simulink model "hydrofoil_sim_unified"  (R2024b)
settings: Solver=VariableStepAuto  StartTime=0.0  StopTime=20  FixedStep=0.05  MaxStep=0.2  RelTol=1e-3
values from neighbouring files (symbols this model uses):
  AfoilA = 0.046    [model_parameters.m]
  AfoilFP = 0.048    [model_parameters.m]
  AfoilFS = 0.048    [model_parameters.m]
  alpha0012 = data0012(:,1)    [model_parameters.m]
  alpha63412wing = data63412wing(:,1)    [model_parameters.m]
  cd0012 = data0012(:,3)    [model_parameters.m]
  cdi63412wing = data63412wing(:,4)    [model_parameters.m]
  cdv63412wing = data63412wing(:,5)    [model_parameters.m]
  cl63412wing = data63412wing(:,3)    [model_parameters.m]
  cm63412wing = data63412wing(:,9)    [model_parameters.m]
  csA = 0.1    [model_parameters.m]
  csF = 0.08    [model_parameters.m]
  deltat = 1/100    (= 0.01)    [model_parameters.m]
  foilA_ARM = [-dxa, dya, dza]    [model_parameters.m]
  foilFP_ARM = [dxf, -dyf, dzf]    [model_parameters.m]
  foilFS_ARM = [dxf, dyf, dzf]    [model_parameters.m]
  g = 9.81    [model_parameters.m]
  LAd = 0.08*pi*(0.8)^3/64    (= 0.0020106192983)    [model_parameters.m]
  LFPd = integral(fpint, foilFP_ARM(2)-0.4, foilFP_ARM(2)+0.4)    [model_parameters.m]
  LFSd = integral(fsint, foilFS_ARM(2)-0.4, foilFS_ARM(2)+0.4)    [model_parameters.m]
  M_RB_1 = inv(M_RB)    [dimensionalize_model.m]    (also in model_parameters.m = M_RB^(-1))
  MAC_A = 0.08    [model_parameters.m]
  MAC_FP = 0.08    [model_parameters.m]
  MAC_FS = 0.08    [model_parameters.m]
  mass = 215    [dimensionalize_model.m]    (also in model_parameters.m)
  propwake = 0.05    [model_parameters.m]
  psd_acc = (9.81*60*1e-6)^2    (= 3.4644996e-07)    [model_parameters.m]
  psd_gyro = (1.222*1e-4)^2    (= 1.493284e-08)    [model_parameters.m]
  r_g = [0; 0; 0]    [dimensionalize_model.m]    (also in model_parameters.m = [xg, yg, zg])
  rho = 1024.8    [model_parameters.m]
  seed_accX = 1324    [model_parameters.m]
  seed_accZ = 1432    [model_parameters.m]
  seed_gps = 4321    [model_parameters.m]
  seed_gyroX = 243251    [model_parameters.m]
  seed_gyroY = 3124234    [model_parameters.m]
  seed_pitch = 7568    [model_parameters.m]
  seed_roll = 35642    [model_parameters.m]
  seed_sonar = 1234    [model_parameters.m]
  setpoint_signals = setpoints.preview    [model_parameters.m]
  sonar_position = [dxf+0.5; 0; -0.1]    [model_parameters.m]
  spanA = 0.76    [model_parameters.m]
  spanFP = 0.76    [model_parameters.m]
  spanFS = 0.76    [model_parameters.m]
  tA = 0.12*0.08    (= 0.0096)    [model_parameters.m]
  tFP = 0.12*0.08    (= 0.0096)    [model_parameters.m]
  tFS = 0.12*0.08    (= 0.0096)    [model_parameters.m]
  usted = 7    [model_parameters.m]
  var_angle = deg2rad(0.2)^2    [model_parameters.m]
  var_gps = 0.05^2    (= 0.0025)    [model_parameters.m]
  var_sonar = 0.002^2    (= 4e-06)    [model_parameters.m]
  wagC1 = 0.165    [model_parameters.m]
  wagC2 = 0.335    [model_parameters.m]
  wage1 = 0.0455*(usted/(MAC_FP/2))    (= 7.9625)    [model_parameters.m]
  wage2 = 0.3*(usted/(MAC_FP/2))    (= 52.5)    [model_parameters.m]
  wave_data = struct('amplitude',0,'omega',0,'wavenumber',0,'phase',0,'direction',0)    [model_parameters.m]
  zpr = dza    (= 0.96)    [model_parameters.m]
undefined symbols (not defined in the file or in its folder): act_lims, actuation_tau, bA, bB, bC, bD, dLTI_array_IDP, dLTI_array_IP, Ka, Klqid, magnitude, PredictionHorizon, set, Ts_reference_preview, V_vals
libraries: mssSimulink x15, mpclib x10, simulink x6, simulink_extras x5, cstblocks x4, matrix_library x3, slpidlib x1
(part 2 of 3)

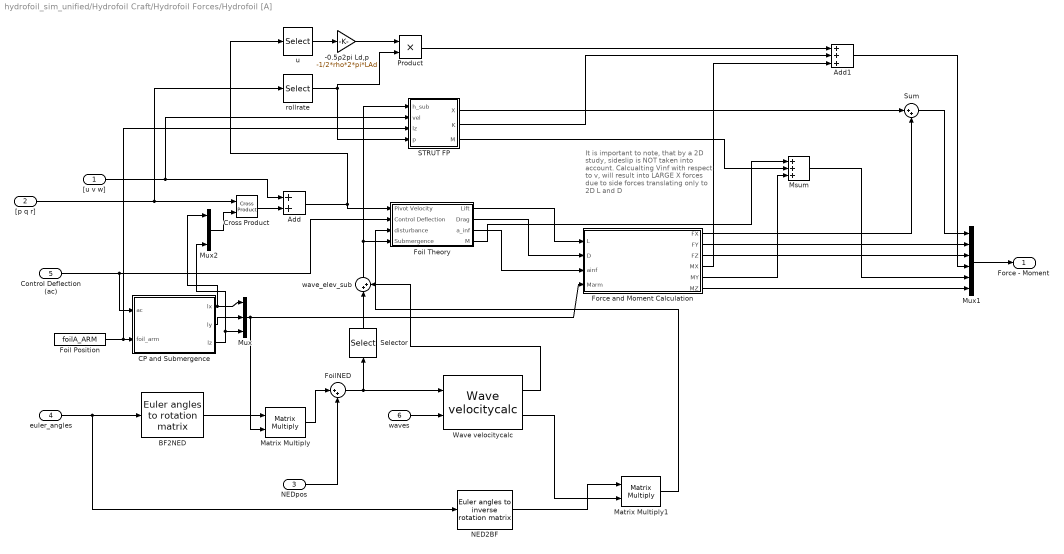
== system hydrofoil_sim_unified/Hydrofoil Craft/Hydrofoil Forces/Hydrofoil [A] ==
  note: It is important to note,
      | that by a 2D study, sideslip
      | is NOT taken into account.
      | Calcualting Vinf with respect
      | to v, will result into LARGE X
      | forces due to side forces translating
      | only to 2D L and D
  "[u v w]" : Inport
  "[p q r]" : Inport  Port=2
  NEDpos : Inport  Port=3
  euler_angles : Inport  Port=4
  Control Deflection (ac) : Inport  Port=5
  waves : Inport  Port=6
  -0.5ρ2pi Ld,p : Gain  Gain=-1/2*rho*2*pi*LAd
  Add : Sum
  Add1 : Sum  Inputs=+++
  BF2NED : mssSimulink/Modelling/Kinematics/Euler angles to rotation matrix
  CP and Submergence : MATLAB Function  TreatAsAtomicUnit=on
  Cross Product : matrix_library/Cross Product
  Foil Position : Constant  Value=foilA_ARM
  Foil Theory : Subsystem
  FoilNED : Sum  Inputs=|++
  Force and Moment Calculation : MATLAB Function  TreatAsAtomicUnit=on
  Matrix Multiply : Product  Multiplication=Matrix(*)
  Matrix Multiply1 : Product  Multiplication=Matrix(*)
  Msum : Sum  Inputs=+++
  Mux : Mux  Inputs=3
  Mux1 : Mux  Inputs=6
  Mux2 : Mux  Inputs=3
  NED2BF : mssSimulink/Modelling/Kinematics/Euler angles to inverse rotation matrix
  Product : Product
  STRUT FP : Subsystem
  Selector : Selector  InputPortWidth=3  IndexOptions=Index vector (dialog)  Indices=[3]  OutputSizes=1
  Sum : Sum  Inputs=|++
  Wave velocitycalc : mssSimulink/Environment/Waves/Wave velocitycalc
  rollrate : Selector  InputPortWidth=3  IndexOptions=Index vector (dialog)  Indices=[1]  OutputSizes=1
  u : Selector  InputPortWidth=3  IndexOptions=Index vector (dialog)  Indices=[1]  OutputSizes=1
  wave_elev_sub : Sum  Inputs=|++
  Force - Moment : Outport
  wires:
  "[u v w]"/1 -> STRUT FP/2(vel), Add/1
  Cross Product/1 -> Add/2
  "[p q r]"/1 -> rollrate/1, Cross Product/1
  Control Deflection (ac)/1 -> Foil Theory/2(Control Deflection), CP and Submergence/1(ac)
  CP and Submergence/1(lx) -> Mux2/1, Mux/1
  CP and Submergence/2(ly) -> Mux/2
  CP and Submergence/3(lz) -> Mux2/3, Mux/3
  Mux/1 -> Matrix Multiply/2, Force and Moment Calculation/4(Marm)
  Force and Moment Calculation/2(FY) -> Mux1/2
  Force and Moment Calculation/3(FZ) -> Mux1/3
  Force and Moment Calculation/6(MZ) -> Mux1/6
  Mux1/1 -> Force - Moment/1
  Foil Position/1 -> STRUT FP/3(lz), CP and Submergence/2(foil_arm)
  euler_angles/1 -> NED2BF/1, BF2NED/1
  Add/1 -> u/1, Foil Theory/1(Pivot Velocity)
  Foil Theory/1(Lift) -> Force and Moment Calculation/1(L)
  Foil Theory/2(Drag) -> Force and Moment Calculation/2(D)
  Foil Theory/3(a_inf) -> Force and Moment Calculation/3(ainf)
  BF2NED/1 -> Matrix Multiply/1
  Matrix Multiply/1 -> FoilNED/1
  NEDpos/1 -> FoilNED/2
  FoilNED/1 -> Wave velocitycalc/1, Selector/1
  Sum/1 -> Mux1/1
  Force and Moment Calculation/1(FX) -> Sum/2
  STRUT FP/1(X) -> Sum/1
  STRUT FP/3(M) -> Msum/2
  Force and Moment Calculation/5(MY) -> Msum/3
  Msum/1 -> Mux1/5
  STRUT FP/2(K) -> Add1/2
  Force and Moment Calculation/4(MX) -> Add1/3
  Add1/1 -> Mux1/4
  Mux2/1 -> Cross Product/2
  rollrate/1 -> Product/2, STRUT FP/4(p)
  -0.5ρ2pi Ld,p/1 -> Product/1
  u/1 -> -0.5ρ2pi Ld,p/1
  Product/1 -> Add1/1
  Wave velocitycalc/1 -> wave_elev_sub/2
  Wave velocitycalc/2 -> Matrix Multiply1/2
  NED2BF/1 -> Matrix Multiply1/1
  wave_elev_sub/1 -> STRUT FP/1(h_sub), Foil Theory/4(Submergence)
  Selector/1 -> wave_elev_sub/1
  waves/1 -> Wave velocitycalc/2
  Matrix Multiply1/1 -> Foil Theory/3(disturbance)
  Foil Theory/4(M) -> Msum/1

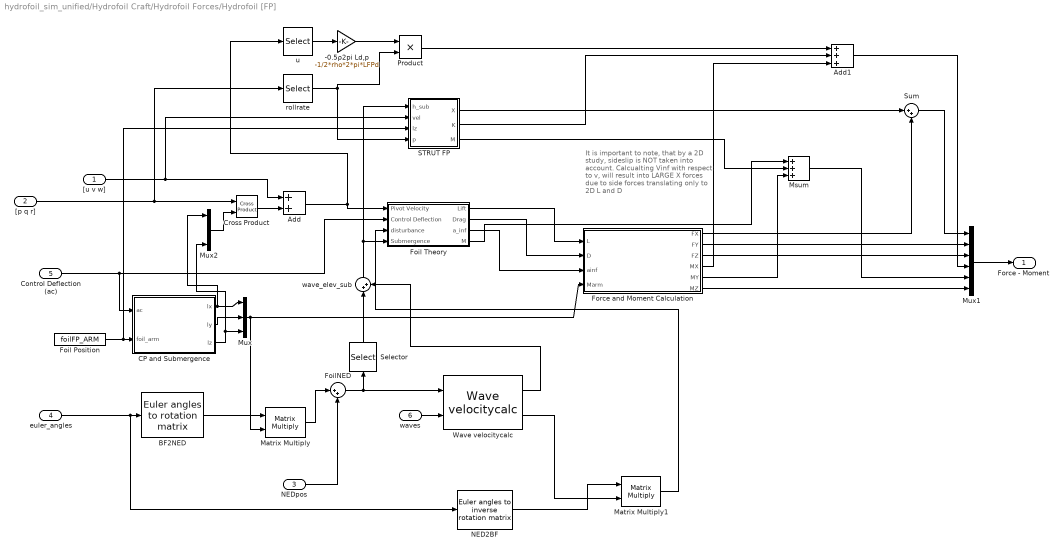
== system hydrofoil_sim_unified/Hydrofoil Craft/Hydrofoil Forces/Hydrofoil [FP] ==
  note: It is important to note,
      | that by a 2D study, sideslip
      | is NOT taken into account.
      | Calcualting Vinf with respect
      | to v, will result into LARGE X
      | forces due to side forces translating
      | only to 2D L and D
  "[u v w]" : Inport
  "[p q r]" : Inport  Port=2
  NEDpos : Inport  Port=3
  euler_angles : Inport  Port=4
  Control Deflection (ac) : Inport  Port=5
  waves : Inport  Port=6
  -0.5ρ2pi Ld,p : Gain  Gain=-1/2*rho*2*pi*LFPd
  Add : Sum
  Add1 : Sum  Inputs=+++
  BF2NED : mssSimulink/Modelling/Kinematics/Euler angles to rotation matrix
  CP and Submergence : MATLAB Function  TreatAsAtomicUnit=on
  Cross Product : matrix_library/Cross Product
  Foil Position : Constant  Value=foilFP_ARM
  Foil Theory : Subsystem
  FoilNED : Sum  Inputs=|++
  Force and Moment Calculation : MATLAB Function  TreatAsAtomicUnit=on
  Matrix Multiply : Product  Multiplication=Matrix(*)
  Matrix Multiply1 : Product  Multiplication=Matrix(*)
  Msum : Sum  Inputs=+++
  Mux : Mux  Inputs=3
  Mux1 : Mux  Inputs=6
  Mux2 : Mux  Inputs=3
  NED2BF : mssSimulink/Modelling/Kinematics/Euler angles to inverse rotation matrix
  Product : Product
  STRUT FP : Subsystem
  Selector : Selector  InputPortWidth=3  IndexOptions=Index vector (dialog)  Indices=[3]  OutputSizes=1
  Sum : Sum  Inputs=|++
  Wave velocitycalc : mssSimulink/Environment/Waves/Wave velocitycalc
  rollrate : Selector  InputPortWidth=3  IndexOptions=Index vector (dialog)  Indices=[1]  OutputSizes=1
  u : Selector  InputPortWidth=3  IndexOptions=Index vector (dialog)  Indices=[1]  OutputSizes=1
  wave_elev_sub : Sum  Inputs=|++
  Force - Moment : Outport
  wires:
  "[u v w]"/1 -> STRUT FP/2(vel), Add/1
  Cross Product/1 -> Add/2
  "[p q r]"/1 -> rollrate/1, Cross Product/1
  Control Deflection (ac)/1 -> Foil Theory/2(Control Deflection), CP and Submergence/1(ac)
  CP and Submergence/1(lx) -> Mux2/1, Mux/1
  CP and Submergence/2(ly) -> Mux/2
  CP and Submergence/3(lz) -> Mux2/3, Mux/3
  Mux/1 -> Matrix Multiply/2, Force and Moment Calculation/4(Marm)
  Force and Moment Calculation/2(FY) -> Mux1/2
  Force and Moment Calculation/3(FZ) -> Mux1/3
  Force and Moment Calculation/6(MZ) -> Mux1/6
  Mux1/1 -> Force - Moment/1
  Foil Position/1 -> STRUT FP/3(lz), CP and Submergence/2(foil_arm)
  euler_angles/1 -> NED2BF/1, BF2NED/1
  Add/1 -> u/1, Foil Theory/1(Pivot Velocity)
  Foil Theory/1(Lift) -> Force and Moment Calculation/1(L)
  Foil Theory/2(Drag) -> Force and Moment Calculation/2(D)
  Foil Theory/3(a_inf) -> Force and Moment Calculation/3(ainf)
  BF2NED/1 -> Matrix Multiply/1
  Matrix Multiply/1 -> FoilNED/1
  NEDpos/1 -> FoilNED/2
  FoilNED/1 -> Wave velocitycalc/1, Selector/1
  Sum/1 -> Mux1/1
  Force and Moment Calculation/1(FX) -> Sum/2
  STRUT FP/1(X) -> Sum/1
  STRUT FP/3(M) -> Msum/2
  Force and Moment Calculation/5(MY) -> Msum/3
  Msum/1 -> Mux1/5
  STRUT FP/2(K) -> Add1/2
  Force and Moment Calculation/4(MX) -> Add1/3
  Add1/1 -> Mux1/4
  Mux2/1 -> Cross Product/2
  rollrate/1 -> Product/2, STRUT FP/4(p)
  -0.5ρ2pi Ld,p/1 -> Product/1
  u/1 -> -0.5ρ2pi Ld,p/1
  Product/1 -> Add1/1
  waves/1 -> Wave velocitycalc/2
  Wave velocitycalc/1 -> wave_elev_sub/2
  NED2BF/1 -> Matrix Multiply1/1
  Wave velocitycalc/2 -> Matrix Multiply1/2
  Selector/1 -> wave_elev_sub/1
  wave_elev_sub/1 -> STRUT FP/1(h_sub), Foil Theory/4(Submergence)
  Matrix Multiply1/1 -> Foil Theory/3(disturbance)
  Foil Theory/4(M) -> Msum/1

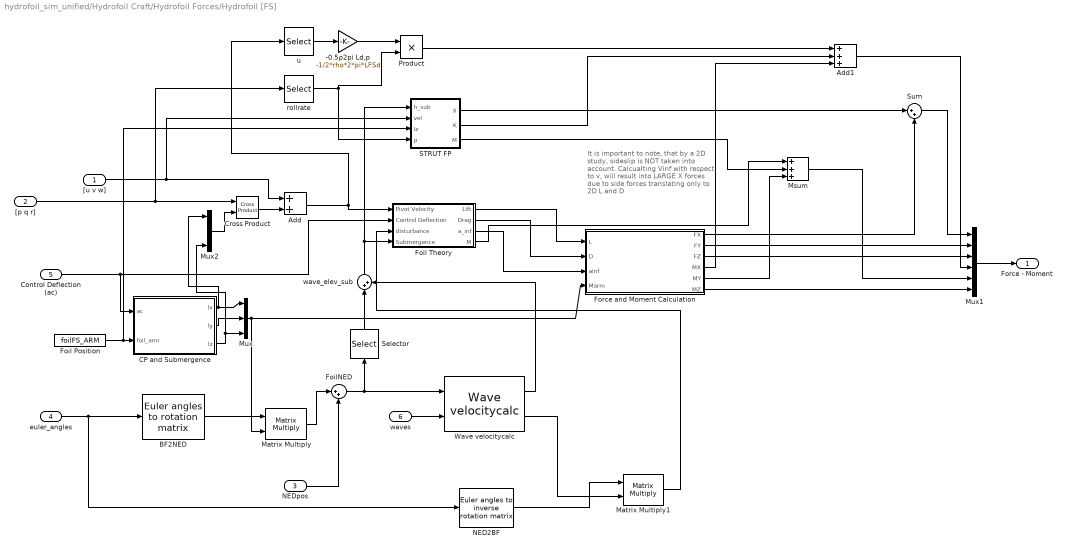
== system hydrofoil_sim_unified/Hydrofoil Craft/Hydrofoil Forces/Hydrofoil [FS] ==
  note: It is important to note,
      | that by a 2D study, sideslip
      | is NOT taken into account.
      | Calcualting Vinf with respect
      | to v, will result into LARGE X
      | forces due to side forces translating
      | only to 2D L and D
  "[u v w]" : Inport
  "[p q r]" : Inport  Port=2
  NEDpos : Inport  Port=3
  euler_angles : Inport  Port=4
  Control Deflection (ac) : Inport  Port=5
  waves : Inport  Port=6
  -0.5ρ2pi Ld,p : Gain  Gain=-1/2*rho*2*pi*LFSd
  Add : Sum
  Add1 : Sum  Inputs=+++
  BF2NED : mssSimulink/Modelling/Kinematics/Euler angles to rotation matrix
  CP and Submergence : MATLAB Function  TreatAsAtomicUnit=on
  Cross Product : matrix_library/Cross Product
  Foil Position : Constant  Value=foilFS_ARM
  Foil Theory : Subsystem
  FoilNED : Sum  Inputs=|++
  Force and Moment Calculation : MATLAB Function  TreatAsAtomicUnit=on
  Matrix Multiply : Product  Multiplication=Matrix(*)
  Matrix Multiply1 : Product  Multiplication=Matrix(*)
  Msum : Sum  Inputs=+++
  Mux : Mux  Inputs=3
  Mux1 : Mux  Inputs=6
  Mux2 : Mux  Inputs=3
  NED2BF : mssSimulink/Modelling/Kinematics/Euler angles to inverse rotation matrix
  Product : Product
  STRUT FP : Subsystem
  Selector : Selector  InputPortWidth=3  IndexOptions=Index vector (dialog)  Indices=[3]  OutputSizes=1
  Sum : Sum  Inputs=|++
  Wave velocitycalc : mssSimulink/Environment/Waves/Wave velocitycalc
  rollrate : Selector  InputPortWidth=3  IndexOptions=Index vector (dialog)  Indices=[1]  OutputSizes=1
  u : Selector  InputPortWidth=3  IndexOptions=Index vector (dialog)  Indices=[1]  OutputSizes=1
  wave_elev_sub : Sum  Inputs=|++
  Force - Moment : Outport
  wires:
  "[u v w]"/1 -> STRUT FP/2(vel), Add/1
  Cross Product/1 -> Add/2
  "[p q r]"/1 -> rollrate/1, Cross Product/1
  Control Deflection (ac)/1 -> Foil Theory/2(Control Deflection), CP and Submergence/1(ac)
  CP and Submergence/1(lx) -> Mux2/1, Mux/1
  CP and Submergence/2(ly) -> Mux/2
  CP and Submergence/3(lz) -> Mux2/3, Mux/3
  Mux/1 -> Matrix Multiply/2, Force and Moment Calculation/4(Marm)
  Force and Moment Calculation/2(FY) -> Mux1/2
  Force and Moment Calculation/3(FZ) -> Mux1/3
  Force and Moment Calculation/6(MZ) -> Mux1/6
  Mux1/1 -> Force - Moment/1
  Foil Position/1 -> STRUT FP/3(lz), CP and Submergence/2(foil_arm)
  euler_angles/1 -> NED2BF/1, BF2NED/1
  Add/1 -> u/1, Foil Theory/1(Pivot Velocity)
  Foil Theory/1(Lift) -> Force and Moment Calculation/1(L)
  Foil Theory/2(Drag) -> Force and Moment Calculation/2(D)
  Foil Theory/3(a_inf) -> Force and Moment Calculation/3(ainf)
  BF2NED/1 -> Matrix Multiply/1
  Matrix Multiply/1 -> FoilNED/1
  NEDpos/1 -> FoilNED/2
  FoilNED/1 -> Selector/1, Wave velocitycalc/1
  Sum/1 -> Mux1/1
  Force and Moment Calculation/1(FX) -> Sum/2
  STRUT FP/1(X) -> Sum/1
  STRUT FP/3(M) -> Msum/2
  Force and Moment Calculation/5(MY) -> Msum/3
  Msum/1 -> Mux1/5
  STRUT FP/2(K) -> Add1/2
  Force and Moment Calculation/4(MX) -> Add1/3
  Add1/1 -> Mux1/4
  Mux2/1 -> Cross Product/2
  rollrate/1 -> Product/2, STRUT FP/4(p)
  -0.5ρ2pi Ld,p/1 -> Product/1
  u/1 -> -0.5ρ2pi Ld,p/1
  Product/1 -> Add1/1
  Wave velocitycalc/1 -> wave_elev_sub/2
  Wave velocitycalc/2 -> Matrix Multiply1/2
  NED2BF/1 -> Matrix Multiply1/1
  Selector/1 -> wave_elev_sub/1
  wave_elev_sub/1 -> STRUT FP/1(h_sub), Foil Theory/4(Submergence)
  waves/1 -> Wave velocitycalc/2
  Matrix Multiply1/1 -> Foil Theory/3(disturbance)
  Foil Theory/4(M) -> Msum/1

== system hydrofoil_sim_unified/sense/sonar/sensor ==
  environment : Inport
  position : Inport  Port=2
  angles : Inport  Port=3
  sonar_pos : Inport  Port=4
  BF2NED : mssSimulink/Modelling/Kinematics/Euler angles to rotation matrix
  Product : Product  Multiplication=Matrix(*)
  Sum : Sum  Inputs=|++
  Sum1 : Sum  Inputs=|++
  Wave velocitycalc : mssSimulink/Environment/Waves/Wave velocitycalc
  get_hs : MATLAB Function  TreatAsAtomicUnit=on
  sonar_height : Outport
  wires:
  environment/1 -> Wave velocitycalc/2
  position/1 -> get_hs/1(positionCG), Sum/1
  angles/1 -> get_hs/2(euler_angles), BF2NED/1
  sonar_pos/1 -> get_hs/3(sonar_position)
  Sum/1 -> Wave velocitycalc/1
  Wave velocitycalc/1 -> Sum1/1
  get_hs/1(h_s) -> Sum1/2
  Sum1/1 -> sonar_height/1
  BF2NED/1 -> Product/1
  get_hs/2(d_s) -> Product/2
  Product/1 -> Sum/2

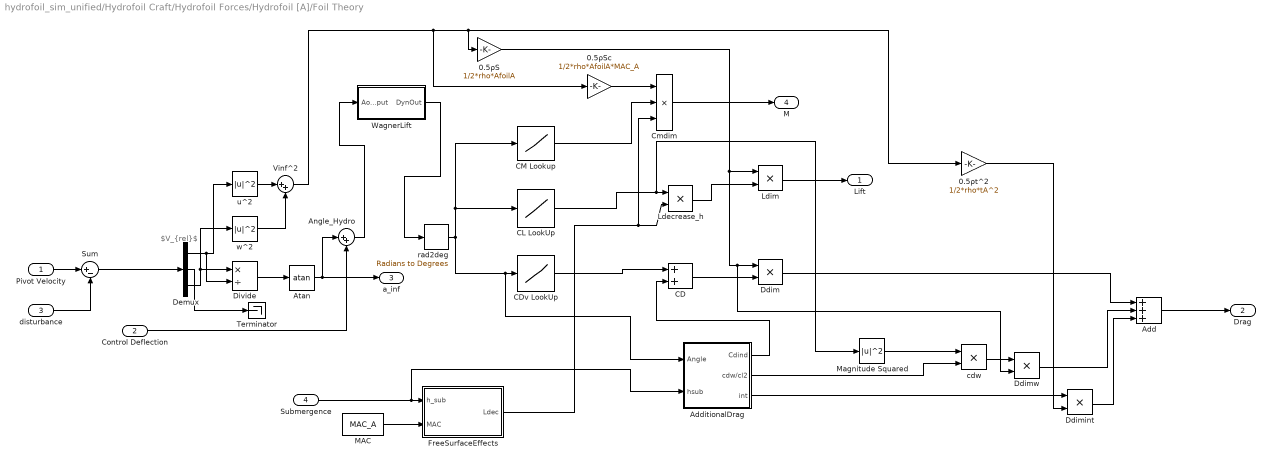
== system hydrofoil_sim_unified/Hydrofoil Craft/Hydrofoil Forces/Hydrofoil [A]/Foil Theory ==
  note: $V_{rel}$
  Pivot Velocity : Inport
  Control Deflection : Inport  Port=2
  disturbance : Inport  Port=3
  Submergence : Inport  Port=4
  0.5ρS : Gain  Gain=1/2*rho*AfoilA
  0.5ρSc : Gain  Gain=1/2*rho*AfoilA*MAC_A
  0.5ρt^2 : Gain  Gain=1/2*rho*tA^2
  Add : Sum  Inputs=+++
  AdditionalDrag : Subsystem
  Angle_Hydro : Sum  Inputs=|++
  Atan : Trigonometry  Operator=atan
  CD : Sum
  CDv LookUp : Lookup_n-D  NumberOfTableDimensions=1  BreakpointsForDimension1=alpha63412wing  Table=cdv63412wing  InternalRulePriority=Speed  RndMeth=Simplest
  CL LookUp : Lookup_n-D  NumberOfTableDimensions=1  BreakpointsForDimension1=alpha63412wing  Table=cl63412wing  InternalRulePriority=Speed  RndMeth=Simplest
  CM Lookup : Lookup_n-D  NumberOfTableDimensions=1  BreakpointsForDimension1=alpha63412wing  Table=cm63412wing  InternalRulePriority=Speed  RndMeth=Simplest
  Cmdim : Product  Inputs=3
  Ddim : Product
  Ddimint : Product
  Ddimw : Product
  Demux : Demux  Outputs=3
  Divide : Product  Inputs=*/
  FreeSurfaceEffects : MATLAB Function  TreatAsAtomicUnit=on
  Ldecrease_h : Product
  Ldim : Product
  MAC : Constant  Value=MAC_A
  Magnitude Squared : Math  Operator=magnitude^2
  Sum : Sum  Inputs=|+-
  Terminator : Terminator
  Vinf^2 : Sum  Inputs=|++
  WagnerLift : Subsystem
  cdw : Product
  rad2deg : simulink_extras/Transformations/Radians to Degrees
  u^2 : Math  Operator=magnitude^2
  w^2 : Math  Operator=magnitude^2
  Lift : Outport
  Drag : Outport  Port=2
  a_inf : Outport  Port=3
  M : Outport  Port=4
  wires:
  rad2deg/1 -> AdditionalDrag/1(Angle), CDv LookUp/1, CM Lookup/1, CL LookUp/1
  Demux/3 -> w^2/1, Divide/1
  Vinf^2/1 -> 0.5ρSc/1, 0.5ρS/1, 0.5ρt^2/1
  w^2/1 -> Vinf^2/2
  Demux/1 -> u^2/1, Divide/2
  Atan/1 -> a_inf/1, Angle_Hydro/1
  0.5ρS/1 -> Ddimw/2, Ddim/1, Ldim/1
  u^2/1 -> Vinf^2/1
  Divide/1 -> Atan/1
  Control Deflection/1 -> Angle_Hydro/2
  Demux/2 -> Terminator/1
  Ldim/1 -> Lift/1
  Sum/1 -> Demux/1
  disturbance/1 -> Sum/2
  Pivot Velocity/1 -> Sum/1
  Submergence/1 -> AdditionalDrag/2(hsub), FreeSurfaceEffects/1(h_sub)
  MAC/1 -> FreeSurfaceEffects/2(MAC)
  FreeSurfaceEffects/1(Ldec) -> Cmdim/3, Ldecrease_h/2
  CL LookUp/1 -> Magnitude Squared/1, Ldecrease_h/1
  Ldecrease_h/1 -> Ldim/2
  CDv LookUp/1 -> CD/1
  CD/1 -> Ddim/2
  AdditionalDrag/1(Cdind) -> CD/2
  Ddim/1 -> Add/1
  Magnitude Squared/1 -> cdw/1
  AdditionalDrag/2(cdw/cl2) -> cdw/2
  cdw/1 -> Ddimw/1
  Ddimw/1 -> Add/2
  AdditionalDrag/3(int) -> Ddimint/1
  Add/1 -> Drag/1
  0.5ρt^2/1 -> Ddimint/2
  Ddimint/1 -> Add/3
  Angle_Hydro/1 -> WagnerLift/1(AoA Input)
  CM Lookup/1 -> Cmdim/2
  0.5ρSc/1 -> Cmdim/1
  Cmdim/1 -> M/1
  WagnerLift/1(DynOut) -> rad2deg/1

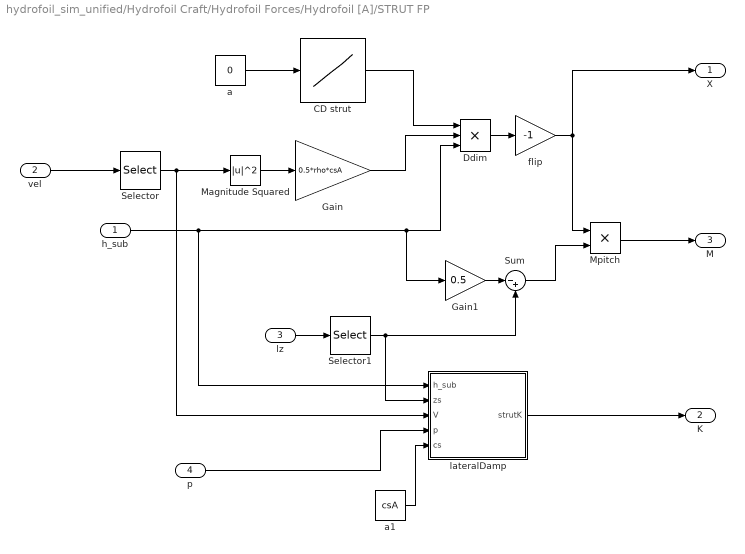
== system hydrofoil_sim_unified/Hydrofoil Craft/Hydrofoil Forces/Hydrofoil [A]/STRUT FP ==
  h_sub : Inport
  vel : Inport  Port=2
  lz : Inport  Port=3
  p : Inport  Port=4
  CD strut : Lookup_n-D  NumberOfTableDimensions=1  BreakpointsForDimension1=alpha0012  Table=cd0012  InternalRulePriority=Speed  RndMeth=Simplest
  Ddim : Product  Inputs=3
  Gain : Gain  Gain=0.5*rho*csA
  Gain1 : Gain  Gain=0.5
  Magnitude Squared : Math  Operator=magnitude^2
  Mpitch : Product
  Selector : Selector  InputPortWidth=3  IndexOptions=Index vector (dialog)  Indices=[1]  OutputSizes=1
  Selector1 : Selector  InputPortWidth=3  IndexOptions=Index vector (dialog)  Indices=[3]  OutputSizes=1
  Sum : Sum  Inputs=|-+
  a : Constant  Value=0
  a1 : Constant  Value=csA
  flip : Gain  Gain=-1
  lateralDamp : MATLAB Function  TreatAsAtomicUnit=on
  X : Outport
  K : Outport  Port=2
  M : Outport  Port=3
  wires:
  vel/1 -> Selector/1
  Selector/1 -> Magnitude Squared/1, lateralDamp/3(V)
  Magnitude Squared/1 -> Gain/1
  a/1 -> CD strut/1
  CD strut/1 -> Ddim/1
  Gain/1 -> Ddim/2
  h_sub/1 -> lateralDamp/1(h_sub), Ddim/3, Gain1/1
  Mpitch/1 -> M/1
  Gain1/1 -> Sum/1
  Sum/1 -> Mpitch/2
  Ddim/1 -> flip/1
  flip/1 -> Mpitch/1, X/1
  lz/1 -> Selector1/1
  Selector1/1 -> lateralDamp/2(zs), Sum/2
  a1/1 -> lateralDamp/5(cs)
  p/1 -> lateralDamp/4(p)
  lateralDamp/1(strutK) -> K/1

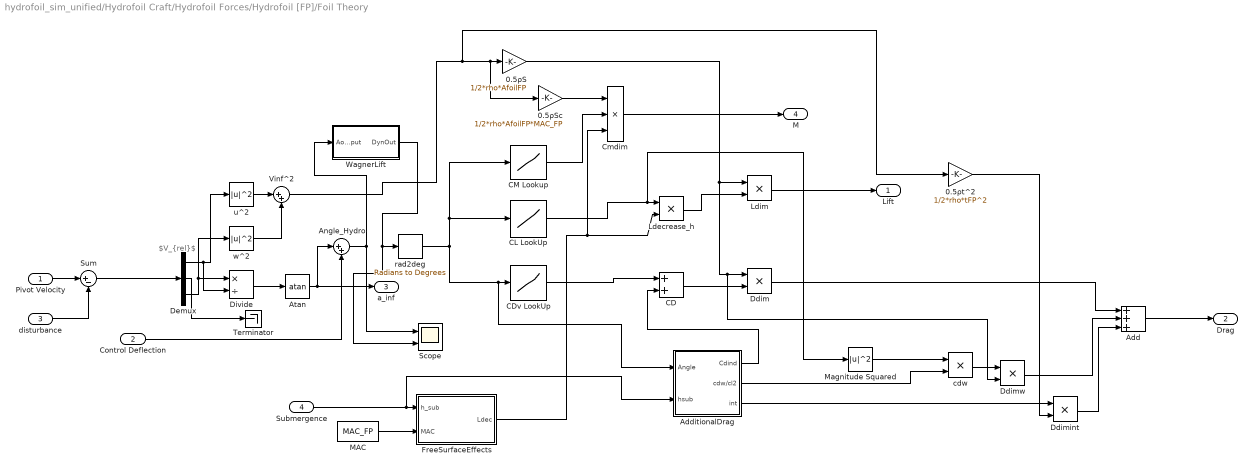
== system hydrofoil_sim_unified/Hydrofoil Craft/Hydrofoil Forces/Hydrofoil [FP]/Foil Theory ==
  note: $V_{rel}$
  Pivot Velocity : Inport
  Control Deflection : Inport  Port=2
  disturbance : Inport  Port=3
  Submergence : Inport  Port=4
  0.5ρS : Gain  Gain=1/2*rho*AfoilFP
  0.5ρSc : Gain  Gain=1/2*rho*AfoilFP*MAC_FP
  0.5ρt^2 : Gain  Gain=1/2*rho*tFP^2
  Add : Sum  Inputs=+++
  AdditionalDrag : Subsystem
  Angle_Hydro : Sum  Inputs=|++
  Atan : Trigonometry  Operator=atan
  CD : Sum
  CDv LookUp : Lookup_n-D  NumberOfTableDimensions=1  BreakpointsForDimension1=alpha63412wing  Table=cdv63412wing  InternalRulePriority=Speed  RndMeth=Simplest
  CL LookUp : Lookup_n-D  NumberOfTableDimensions=1  BreakpointsForDimension1=alpha63412wing  Table=cl63412wing  InternalRulePriority=Speed  RndMeth=Simplest
  CM Lookup : Lookup_n-D  NumberOfTableDimensions=1  BreakpointsForDimension1=alpha63412wing  Table=cm63412wing  InternalRulePriority=Speed  RndMeth=Simplest
  Cmdim : Product  Inputs=3
  Ddim : Product
  Ddimint : Product
  Ddimw : Product
  Demux : Demux  Outputs=3
  Divide : Product  Inputs=*/
  FreeSurfaceEffects : MATLAB Function  TreatAsAtomicUnit=on
  Ldecrease_h : Product
  Ldim : Product
  MAC : Constant  Value=MAC_FP
  Magnitude Squared : Math  Operator=magnitude^2
  Scope : Scope  NumInputPorts=2
  Sum : Sum  Inputs=|+-
  Terminator : Terminator
  Vinf^2 : Sum  Inputs=|++
  WagnerLift : Subsystem
  cdw : Product
  rad2deg : simulink_extras/Transformations/Radians to Degrees
  u^2 : Math  Operator=magnitude^2
  w^2 : Math  Operator=magnitude^2
  Lift : Outport
  Drag : Outport  Port=2
  a_inf : Outport  Port=3
  M : Outport  Port=4
  wires:
  rad2deg/1 -> AdditionalDrag/1(Angle), CDv LookUp/1, CM Lookup/1, CL LookUp/1
  Demux/3 -> w^2/1, Divide/1
  Vinf^2/1 -> 0.5ρt^2/1, 0.5ρSc/1, 0.5ρS/1
  w^2/1 -> Vinf^2/2
  Demux/1 -> u^2/1, Divide/2
  Atan/1 -> a_inf/1, Angle_Hydro/1
  0.5ρS/1 -> Ddimw/2, Ddim/1, Ldim/1
  u^2/1 -> Vinf^2/1
  Divide/1 -> Atan/1
  Control Deflection/1 -> Angle_Hydro/2
  Demux/2 -> Terminator/1
  Sum/1 -> Demux/1
  disturbance/1 -> Sum/2
  Pivot Velocity/1 -> Sum/1
  Submergence/1 -> AdditionalDrag/2(hsub), FreeSurfaceEffects/1(h_sub)
  MAC/1 -> FreeSurfaceEffects/2(MAC)
  FreeSurfaceEffects/1(Ldec) -> Cmdim/3, Ldecrease_h/2
  CL LookUp/1 -> Magnitude Squared/1, Ldecrease_h/1
  Ldecrease_h/1 -> Ldim/2
  CDv LookUp/1 -> CD/1
  CD/1 -> Ddim/2
  AdditionalDrag/1(Cdind) -> CD/2
  Ddim/1 -> Add/1
  Magnitude Squared/1 -> cdw/1
  AdditionalDrag/2(cdw/cl2) -> cdw/2
  cdw/1 -> Ddimw/1
  Ddimw/1 -> Add/2
  AdditionalDrag/3(int) -> Ddimint/1
  Add/1 -> Drag/1
  0.5ρt^2/1 -> Ddimint/2
  Ddimint/1 -> Add/3
  Ldim/1 -> Lift/1
  Angle_Hydro/1 -> WagnerLift/1(AoA Input), Scope/1
  0.5ρSc/1 -> Cmdim/1
  CM Lookup/1 -> Cmdim/2
  Cmdim/1 -> M/1
  WagnerLift/1(DynOut) -> Scope/2, rad2deg/1

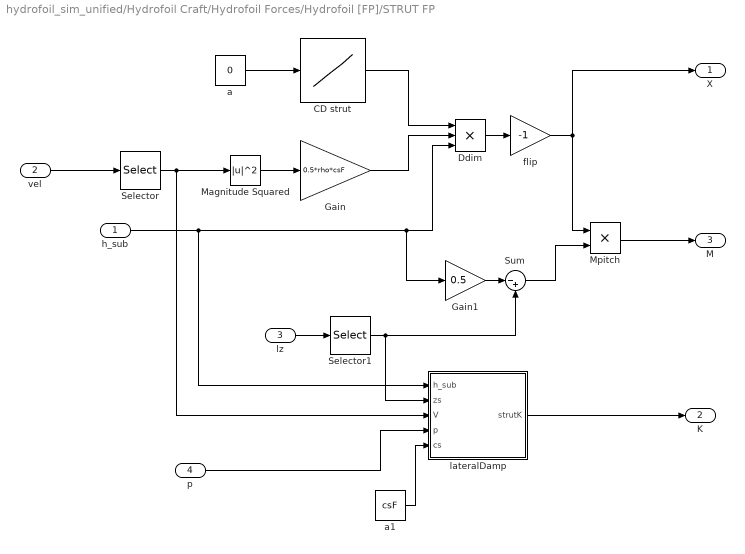
== system hydrofoil_sim_unified/Hydrofoil Craft/Hydrofoil Forces/Hydrofoil [FP]/STRUT FP ==
  h_sub : Inport
  vel : Inport  Port=2
  lz : Inport  Port=3
  p : Inport  Port=4
  CD strut : Lookup_n-D  NumberOfTableDimensions=1  BreakpointsForDimension1=alpha0012  Table=cd0012  InternalRulePriority=Speed  RndMeth=Simplest
  Ddim : Product  Inputs=3
  Gain : Gain  Gain=0.5*rho*csF
  Gain1 : Gain  Gain=0.5
  Magnitude Squared : Math  Operator=magnitude^2
  Mpitch : Product
  Selector : Selector  InputPortWidth=3  IndexOptions=Index vector (dialog)  Indices=[1]  OutputSizes=1
  Selector1 : Selector  InputPortWidth=3  IndexOptions=Index vector (dialog)  Indices=[3]  OutputSizes=1
  Sum : Sum  Inputs=|-+
  a : Constant  Value=0
  a1 : Constant  Value=csF
  flip : Gain  Gain=-1
  lateralDamp : MATLAB Function  TreatAsAtomicUnit=on
  X : Outport
  K : Outport  Port=2
  M : Outport  Port=3
  wires:
  vel/1 -> Selector/1
  Selector/1 -> Magnitude Squared/1, lateralDamp/3(V)
  Magnitude Squared/1 -> Gain/1
  a/1 -> CD strut/1
  CD strut/1 -> Ddim/1
  Gain/1 -> Ddim/2
  h_sub/1 -> lateralDamp/1(h_sub), Ddim/3, Gain1/1
  Mpitch/1 -> M/1
  Gain1/1 -> Sum/1
  Sum/1 -> Mpitch/2
  Ddim/1 -> flip/1
  flip/1 -> Mpitch/1, X/1
  lz/1 -> Selector1/1
  Selector1/1 -> lateralDamp/2(zs), Sum/2
  a1/1 -> lateralDamp/5(cs)
  p/1 -> lateralDamp/4(p)
  lateralDamp/1(strutK) -> K/1

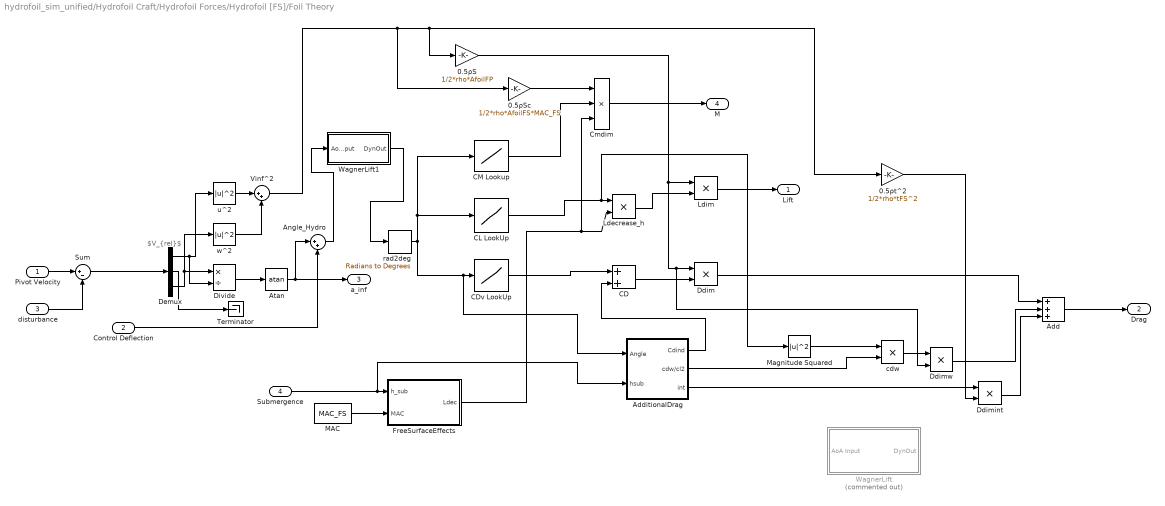
== system hydrofoil_sim_unified/Hydrofoil Craft/Hydrofoil Forces/Hydrofoil [FS]/Foil Theory ==
  note: $V_{rel}$
  Pivot Velocity : Inport
  Control Deflection : Inport  Port=2
  disturbance : Inport  Port=3
  Submergence : Inport  Port=4
  0.5ρS : Gain  Gain=1/2*rho*AfoilFP
  0.5ρSc : Gain  Gain=1/2*rho*AfoilFS*MAC_FS
  0.5ρt^2 : Gain  Gain=1/2*rho*tFS^2
  Add : Sum  Inputs=+++
  AdditionalDrag : Subsystem
  Angle_Hydro : Sum  Inputs=|++
  Atan : Trigonometry  Operator=atan
  CD : Sum
  CDv LookUp : Lookup_n-D  NumberOfTableDimensions=1  BreakpointsForDimension1=alpha63412wing  Table=cdv63412wing  InternalRulePriority=Speed  RndMeth=Simplest
  CL LookUp : Lookup_n-D  NumberOfTableDimensions=1  BreakpointsForDimension1=alpha63412wing  Table=cl63412wing  InternalRulePriority=Speed  RndMeth=Simplest
  CM Lookup : Lookup_n-D  NumberOfTableDimensions=1  BreakpointsForDimension1=alpha63412wing  Table=cm63412wing  InternalRulePriority=Speed  RndMeth=Simplest
  Cmdim : Product  Inputs=3
  Ddim : Product
  Ddimint : Product
  Ddimw : Product
  Demux : Demux  Outputs=3
  Divide : Product  Inputs=*/
  FreeSurfaceEffects : MATLAB Function  TreatAsAtomicUnit=on
  Ldecrease_h : Product
  Ldim : Product
  MAC : Constant  Value=MAC_FS
  Magnitude Squared : Math  Operator=magnitude^2
  Sum : Sum  Inputs=|+-
  Terminator : Terminator
  Vinf^2 : Sum  Inputs=|++
  WagnerLift : Subsystem  Commented=on
  WagnerLift1 : Subsystem
  cdw : Product
  rad2deg : simulink_extras/Transformations/Radians to Degrees
  u^2 : Math  Operator=magnitude^2
  w^2 : Math  Operator=magnitude^2
  Lift : Outport
  Drag : Outport  Port=2
  a_inf : Outport  Port=3
  M : Outport  Port=4
  wires:
  rad2deg/1 -> AdditionalDrag/1(Angle), CDv LookUp/1, CM Lookup/1, CL LookUp/1
  Demux/3 -> w^2/1, Divide/1
  Vinf^2/1 -> 0.5ρSc/1, 0.5ρS/1, 0.5ρt^2/1
  w^2/1 -> Vinf^2/2
  Demux/1 -> u^2/1, Divide/2
  Atan/1 -> a_inf/1, Angle_Hydro/1
  0.5ρS/1 -> Ddimw/2, Ddim/1, Ldim/1
  u^2/1 -> Vinf^2/1
  Divide/1 -> Atan/1
  Control Deflection/1 -> Angle_Hydro/2
  Demux/2 -> Terminator/1
  Ldim/1 -> Lift/1
  Sum/1 -> Demux/1
  disturbance/1 -> Sum/2
  Pivot Velocity/1 -> Sum/1
  Submergence/1 -> AdditionalDrag/2(hsub), FreeSurfaceEffects/1(h_sub)
  MAC/1 -> FreeSurfaceEffects/2(MAC)
  FreeSurfaceEffects/1(Ldec) -> Cmdim/3, Ldecrease_h/2
  CL LookUp/1 -> Magnitude Squared/1, Ldecrease_h/1
  Ldecrease_h/1 -> Ldim/2
  CDv LookUp/1 -> CD/1
  CD/1 -> Ddim/2
  AdditionalDrag/1(Cdind) -> CD/2
  Ddim/1 -> Add/1
  Magnitude Squared/1 -> cdw/1
  AdditionalDrag/2(cdw/cl2) -> cdw/2
  cdw/1 -> Ddimw/1
  Ddimw/1 -> Add/2
  AdditionalDrag/3(int) -> Ddimint/1
  Add/1 -> Drag/1
  0.5ρt^2/1 -> Ddimint/2
  Ddimint/1 -> Add/3
  Angle_Hydro/1 -> WagnerLift1/1(AoA Input)
  Cmdim/1 -> M/1
  0.5ρSc/1 -> Cmdim/1
  CM Lookup/1 -> Cmdim/2
  WagnerLift1/1(DynOut) -> rad2deg/1

== system hydrofoil_sim_unified/Hydrofoil Craft/Hydrofoil Forces/Hydrofoil [FS]/STRUT FP ==
  h_sub : Inport
  vel : Inport  Port=2
  lz : Inport  Port=3
  p : Inport  Port=4
  CD strut : Lookup_n-D  NumberOfTableDimensions=1  BreakpointsForDimension1=alpha0012  Table=cd0012  InternalRulePriority=Speed  RndMeth=Simplest
  Ddim : Product  Inputs=3
  Gain : Gain  Gain=0.5*rho*csF
  Gain1 : Gain  Gain=0.5
  Magnitude Squared : Math  Operator=magnitude^2
  Mpitch : Product
  Selector : Selector  InputPortWidth=3  IndexOptions=Index vector (dialog)  Indices=[1]  OutputSizes=1
  Selector1 : Selector  InputPortWidth=3  IndexOptions=Index vector (dialog)  Indices=[3]  OutputSizes=1
  Sum : Sum  Inputs=|-+
  a : Constant  Value=0
  a1 : Constant  Value=csF
  flip : Gain  Gain=-1
  lateralDamp : MATLAB Function  TreatAsAtomicUnit=on
  X : Outport
  K : Outport  Port=2
  M : Outport  Port=3
  wires:
  vel/1 -> Selector/1
  Selector/1 -> Magnitude Squared/1, lateralDamp/3(V)
  Magnitude Squared/1 -> Gain/1
  a/1 -> CD strut/1
  CD strut/1 -> Ddim/1
  Gain/1 -> Ddim/2
  h_sub/1 -> lateralDamp/1(h_sub), Ddim/3, Gain1/1
  Mpitch/1 -> M/1
  Gain1/1 -> Sum/1
  Sum/1 -> Mpitch/2
  Ddim/1 -> flip/1
  flip/1 -> Mpitch/1, X/1
  lz/1 -> Selector1/1
  Selector1/1 -> lateralDamp/2(zs), Sum/2
  a1/1 -> lateralDamp/5(cs)
  p/1 -> lateralDamp/4(p)
  lateralDamp/1(strutK) -> K/1

== system hydrofoil_sim_unified/Hydrofoil Craft/Hydrofoil Forces/Hydrofoil [A]/Foil Theory/AdditionalDrag ==
  Angle : Inport
  hsub : Inport  Port=2
  Additional Drag : MATLAB Function  TreatAsAtomicUnit=on
  CD induced : Lookup_n-D  NumberOfTableDimensions=1  BreakpointsForDimension1=alpha63412wing  Table=cdi63412wing  InternalRulePriority=Speed  RndMeth=Simplest
  c : Constant  Value=MAC_A
  span : Constant  Value=spanA
  t : Constant  Value=tA
  Cdind : Outport
  cdw/cl2 : Outport  Port=2
  int : Outport  Port=3
  wires:
  Angle/1 -> CD induced/1
  CD induced/1 -> Additional Drag/1(cdind)
  Additional Drag/1(dinc) -> Cdind/1
  span/1 -> Additional Drag/2(span)
  hsub/1 -> Additional Drag/3(hsub)
  t/1 -> Additional Drag/4(t)
  c/1 -> Additional Drag/5(c)
  Additional Drag/2(cdw) -> cdw/cl2/1
  Additional Drag/3(cdint) -> int/1

== system hydrofoil_sim_unified/Hydrofoil Craft/Hydrofoil Forces/Hydrofoil [A]/Foil Theory/WagnerLift ==
  AoA Input : Inport
  Add : Sum  Inputs=+++
  Add1 : Sum
  Gain : Gain  Gain=0.5
  Product : Product
  Product1 : Product
  init_dynamic : Step  Time=0.7  SampleTime=0
  level_model : Step  Time=0.7  Before=1  After=0  SampleTime=0
  wagn1 : TransferFcn  Numerator=[wagC1*wage1]  Denominator=[1 wage1]
  wagn2 : TransferFcn  Numerator=[wagC2*wage2]  Denominator=[1 wage2]
  DynOut : Outport
  wires:
  wagn1/1 -> Add/1
  AoA Input/1 -> Product1/2, wagn1/1, wagn2/1, Gain/1  "input"
  wagn2/1 -> Add/2
  Gain/1 -> Add/3
  Add1/1 -> DynOut/1  "dynout"
  init_dynamic/1 -> Product/2
  Add/1 -> Product/1
  level_model/1 -> Product1/1
  Product1/1 -> Add1/1
  Product/1 -> Add1/2

== system hydrofoil_sim_unified/Hydrofoil Craft/Hydrofoil Forces/Hydrofoil [FP]/Foil Theory/AdditionalDrag ==
  Angle : Inport
  hsub : Inport  Port=2
  Additional Drag : MATLAB Function  TreatAsAtomicUnit=on
  CD induced : Lookup_n-D  NumberOfTableDimensions=1  BreakpointsForDimension1=alpha63412wing  Table=cdi63412wing  InternalRulePriority=Speed  RndMeth=Simplest
  c : Constant  Value=MAC_FP
  span : Constant  Value=spanFP
  t : Constant  Value=tFP
  Cdind : Outport
  cdw/cl2 : Outport  Port=2
  int : Outport  Port=3
  wires:
  Angle/1 -> CD induced/1
  CD induced/1 -> Additional Drag/1(cdind)
  Additional Drag/1(dinc) -> Cdind/1
  span/1 -> Additional Drag/2(span)
  hsub/1 -> Additional Drag/3(hsub)
  t/1 -> Additional Drag/4(t)
  c/1 -> Additional Drag/5(c)
  Additional Drag/2(cdw) -> cdw/cl2/1
  Additional Drag/3(cdint) -> int/1

== system hydrofoil_sim_unified/Hydrofoil Craft/Hydrofoil Forces/Hydrofoil [FP]/Foil Theory/WagnerLift ==
  AoA Input : Inport
  Add : Sum  Inputs=+++
  Add1 : Sum
  Gain : Gain  Gain=0.5
  Product : Product
  Product1 : Product
  init_dynamic : Step  Time=0.7  SampleTime=0
  level_model : Step  Time=0.7  Before=1  After=0  SampleTime=0
  wagn1 : TransferFcn  Numerator=[wagC1*wage1]  Denominator=[1 wage1]
  wagn2 : TransferFcn  Numerator=[wagC2*wage2]  Denominator=[1 wage2]
  DynOut : Outport
  wires:
  wagn1/1 -> Add/1
  AoA Input/1 -> Product1/2, wagn1/1, wagn2/1, Gain/1  "input"
  wagn2/1 -> Add/2
  Gain/1 -> Add/3
  Add1/1 -> DynOut/1  "dynout"
  init_dynamic/1 -> Product/2
  Add/1 -> Product/1
  level_model/1 -> Product1/1
  Product1/1 -> Add1/1
  Product/1 -> Add1/2

== system hydrofoil_sim_unified/Hydrofoil Craft/Hydrofoil Forces/Hydrofoil [FS]/Foil Theory/AdditionalDrag ==
  Angle : Inport
  hsub : Inport  Port=2
  Additional Drag : MATLAB Function  TreatAsAtomicUnit=on
  CD induced : Lookup_n-D  NumberOfTableDimensions=1  BreakpointsForDimension1=alpha63412wing  Table=cdi63412wing  InternalRulePriority=Speed  RndMeth=Simplest
  c : Constant  Value=MAC_FS
  span : Constant  Value=spanFS
  t : Constant  Value=tFS
  Cdind : Outport
  cdw/cl2 : Outport  Port=2
  int : Outport  Port=3
  wires:
  Angle/1 -> CD induced/1
  CD induced/1 -> Additional Drag/1(cdind)
  Additional Drag/1(dinc) -> Cdind/1
  span/1 -> Additional Drag/2(span)
  hsub/1 -> Additional Drag/3(hsub)
  t/1 -> Additional Drag/4(t)
  c/1 -> Additional Drag/5(c)
  Additional Drag/2(cdw) -> cdw/cl2/1
  Additional Drag/3(cdint) -> int/1

== system hydrofoil_sim_unified/Hydrofoil Craft/Hydrofoil Forces/Hydrofoil [FS]/Foil Theory/WagnerLift ==
  AoA Input : Inport
  Add : Sum  Inputs=+++
  Gain : Gain  Gain=0.5
  wagn1 : TransferFcn  Numerator=[wagC1*wage1]  Denominator=[1 wage1]
  wagn2 : TransferFcn  Numerator=[wagC2*wage2]  Denominator=[1 wage2]
  DynOut : Outport
  wires:
  wagn1/1 -> Add/1
  AoA Input/1 -> wagn2/1, Gain/1, wagn1/1
  wagn2/1 -> Add/2
  Gain/1 -> Add/3
  Add/1 -> DynOut/1

== system hydrofoil_sim_unified/Hydrofoil Craft/Hydrofoil Forces/Hydrofoil [FS]/Foil Theory/WagnerLift1 ==
  AoA Input : Inport
  Add : Sum  Inputs=+++
  Add1 : Sum
  Gain : Gain  Gain=0.5
  Product : Product
  Product1 : Product
  init_dynamic : Step  Time=0.7  SampleTime=0
  level_model : Step  Time=0.7  Before=1  After=0  SampleTime=0
  wagn1 : TransferFcn  Numerator=[wagC1*wage1]  Denominator=[1 wage1]
  wagn2 : TransferFcn  Numerator=[wagC2*wage2]  Denominator=[1 wage2]
  DynOut : Outport
  wires:
  wagn1/1 -> Add/1
  AoA Input/1 -> Product1/2, wagn1/1, wagn2/1, Gain/1  "input"
  wagn2/1 -> Add/2
  Gain/1 -> Add/3
  Add1/1 -> DynOut/1  "dynout"
  init_dynamic/1 -> Product/2
  Add/1 -> Product/1
  level_model/1 -> Product1/1
  Product1/1 -> Add1/1
  Product/1 -> Add1/2

== matlab function hydrofoil_sim_unified/Hydrofoil Craft/Hydrofoil Forces/Hydrofoil [A]/Foil Theory/FreeSurfaceEffects ==
  data: Ldec output; h_sub input; MAC input
function Ldec  = fcn(h_sub, MAC)

Ldec = 1 - 0.422*exp(-1.454*(h_sub/MAC));

== matlab function hydrofoil_sim_unified/Hydrofoil Craft/Hydrofoil Forces/Hydrofoil [FS]/CP and Submergence ==
  data: lx output; ly output; ac input; lz output; foil_arm input
function [lx,ly,lz] = CP_HSF(ac, foil_arm)
% This function will calculate the moment arm for the center of 
% pressure of a hydrofoil based on control deflection. 
% Used when the pivot point is different from the center of pressure, and
% set to the original foil CP defined in the params otherwise.



lx = foil_arm(1);
ly = foil_arm(2);
lz = foil_arm(3);

== matlab function hydrofoil_sim_unified/Hydrofoil Craft/EOM/CRB MATRIX ==
  data: C output; nu input; M_RB parameter
% function CRB = CRBmatrix(uvw, pqr, mass, InertiaTensor, CG)
% 
% SMAT = @(x) [0 -x(3) x(2);
%             x(3) 0 -x(1);
%             -x(2) x(1) 0];
% CRB = [zeros(3,3), -mass*SMAT(uvw)-mass*SMAT(pqr)*SMAT(CG);
%         -mass*SMAT(uvw)+mass*SMAT(CG)*SMAT(pqr), -SMAT(InertiaTensor*pqr)];


function C = m2c(nu, M_RB)
M = M_RB;
% C = m2c(M,nu) computes the Coriolis-centripetal matrix C(nu) from the
% the system inertia matrix M > 0 for varying velocity nu. 
% If M is a 6x6 matrix and nu = [u, v, w, p, q, r]', the output is a 6x6 C matrix
% If M is a 3x3 matrix and nu = [u, v, r]', the output is a 3x3 C matrix.
%
% Examples: CRB = m2c(MRB,nu)     
%           CA  = m2c(MA, nu)
% Output:
%  C:  Coriolis-centripetal matrix C = C(nu) 
%
% Inputs:
%  M:  6x6 or 3x3 rigid-body MRB or added mass MA system marix 
%  nu: nu = [u, v, w, p, q, r]' or nu = [u, v, r]'
%
% The Coriolis and centripetal matrix depends on nu1 = [u,v,w]' and nu2 =
% [p,q,r]' as shown in Fossen (2021, Theorem 3.2). Alternatively, the matrix 
% CRB = CRB(nu2) can be computed using 
% 
% [MRB,CRB] = rbody(m,R44,R55,R66,nu2,r_bp) 
%
% which only requires the angular velocity vector nu2 = [p,q,r]'. This is 
% known as the linear velocity-independent representation.
%
% Author:    Thor I. Fossen
% Date:      14 Jun 2001
% Revisions: 26 Jun 2002, M21 = M12 is corrected to M12'
%            10 Jan 2004, the computation of C(nu) is generalized to a 
%                         nonsymmetric M > 0 (experimental data)
%            22 Oct 2020, generalized to accept 3-DOF horizontal-plane models
%            24 Apr 2021, updated the documentation

Smtrx = @(x) [0 -x(3) x(2);
             x(3) 0 -x(1);
            -x(2) x(1) 0];

M = 0.5 * (M + M');      % symmetrization of the inertia matrix

if (length(nu) == 6)     % 6-DOF model
     
    M11 = M(1:3,1:3);
    M12 = M(1:3,4:6);
    M21 = M12';
    M22 = M(4:6,4:6);

    nu1 = nu(1:3);
    nu2 = nu(4:6);
    nu1_dot = M11 * nu1 + M12 * nu2;
    nu2_dot = M21 * nu1 + M22 * nu2;

    C = [  zeros(3,3)      -Smtrx(nu1_dot)
          -Smtrx(nu1_dot)  -Smtrx(nu2_dot) ]; % 3.46 from T.I Fossen Handbook
    
else   % 3-DOF model (surge, sway and yaw)
    
    C = [ 0                          0            -M(2,2)*nu(2)-M(2,3)*nu(3)
          0                          0             M(1,1)*nu(1)
          M(2,2)*nu(2)+M(2,3)*nu(3) -M(1,1)*nu(1)  0                      ];
    
end

== matlab function hydrofoil_sim_unified/Hydrofoil Craft/Hydrofoil Forces/Hydrofoil [FP]/Foil Theory/FreeSurfaceEffects ==
  data: Ldec output; h_sub input; MAC input
function Ldec  = fcn(h_sub, MAC)

Ldec = 1 - 0.422*exp(-1.454*(h_sub/MAC));

== matlab function hydrofoil_sim_unified/Hydrofoil Craft/Kinematics Equations ==
  data: euler_angles input size=3; uvw input size=3; pos_rates output size=3; pqr input size=3; euler_ang_rates output size=3
function [pos_rates, euler_ang_rates]= Kinematics(euler_angles, uvw, pqr)
    
phi = euler_angles(1);
theta = euler_angles(2);
psy = euler_angles(3);

DCM = [cos(psy)*cos(theta), -sin(psy)*cos(phi)+cos(psy)*sin(theta)*sin(phi), sin(psy)*sin(phi)+cos(psy)*cos(phi)*sin(theta);
    sin(psy)*cos(theta), cos(psy)*cos(phi)+sin(phi)*sin(theta)*sin(psy), -cos(psy)*sin(phi)+sin(theta)*sin(psy)*cos(phi);
    -sin(theta), sin(phi)*cos(theta), cos(theta)*cos(phi)];


attitudeMatrix = [1 sin(phi)*tan(theta) cos(phi)*tan(theta);
                  0 cos(phi) -sin(phi);
                  0 sin(phi)/cos(theta) cos(phi)/cos(theta)];

euler_ang_rates = attitudeMatrix*pqr;

pos_rates = DCM*uvw;

== matlab function hydrofoil_sim_unified/Hydrofoil Craft/Hydrofoil Forces/Hydrofoil [FS]/Foil Theory/AdditionalDrag/Additional Drag ==
  data: cdind input; dinc output; span input; hsub input; t input; c input; cdw output; cdint output; usted parameter
function [dinc, cdw, cdint]   = addedDrag(cdind, span, hsub, t, c, usted)

%V = 7m/s not very correct in general 
hsub = abs(hsub);
dinc = (2-(33*(hsub/span)^(3/2))/(33*(hsub/span)^(3/2)+1))*cdind;
frh = usted/sqrt(9.81*hsub);
cdw = 1/(2*frh^2)*(c/hsub)*exp(-2/frh^2);
cdint = 0.75*(t/c)-0.0003*(t/c)^(-2);

== matlab function hydrofoil_sim_unified/Controller [Variant]/LQI-SW/Discrete LQRi ==
  settings: updateMethod=DISCRETE
  data: reference input; states input; control_input output; u_trim input; Klqid parameter; Ka parameter; act_lims parameter
function control_input  = LQRi_discrete(reference, states,  u_trim, Klqid, Ka, act_lims)

% LQRi with internal sample-and-hold behavior
% Inputs:
%   u_ref   - feedforward/reference input
%   z_ref   - reference for tracking
%   y       - measured outputs (vector)
%   t       - current simulation time

% Parameters
T_s = 0.1;  % controller sample time

% Persistent variables
persistent xI_z xI_phi xI_theta
persistent last_update_time u_hold u_c

if isempty(last_update_time)
    xI_z = 0; xI_phi = 0; xI_theta = 0;
    last_update_time = -inf;
    u_c = zeros(3,1);
    u_hold = zeros(3,1);
end


states = states-reference;
% --- Tracking Errors ---
e_z = states(1);
e_phi = states(2);    
e_theta = states(3);  

% --- Integrate Error ---

xI_z = xI_z + T_s * e_z + T_s*Ka(1,:)*(u_hold-u_c);
xI_phi = xI_phi + T_s * e_phi + T_s*Ka(2,:)*(u_hold-u_c);
xI_theta = xI_theta + T_s * e_theta + T_s*Ka(3,:)*(u_hold-u_c);

% --- Control Law ---
x_aug = [states; xI_z; xI_phi; xI_theta];

% Define gain K externally or inline
K = Klqid;  


% Compute control
u_c = u_trim - K * x_aug;

% this alone is saturation
u_hold = min(max(u_c, act_lims(:,1)), act_lims(:,2)); 



% --- Output ZOH value ---
control_input = u_hold;

== matlab function hydrofoil_sim_unified/Hydrofoil Craft/Hydrofoil Forces/Hydrofoil [FS]/Foil Theory/FreeSurfaceEffects ==
  data: Ldec output; h_sub input; MAC input
function Ldec  = fcn(h_sub, MAC)

Ldec = 1 - 0.422*exp(-1.454*(h_sub/MAC));

== matlab function hydrofoil_sim_unified/Hydrofoil Craft/Hydrofoil Forces/Hydrofoil [A]/Force and Moment Calculation ==
  data: L input; D input; FX output; ainf input; FY output; FZ output; Marm input; MX output; MY output; MZ output
function [FX, FY, FZ, MX, MY, MZ] = HydrodynamicForces(L, D, ainf, Marm)


%%%%%%%%% ----------------- %%%%%%%%

% Vrel is :
% u+qz-ry  
% v+rx-pz
% w+py-qx

%Inflow velocity is this vector's magnitude, however, in 2D analysis,
%considering the y direction velocity will lead to issues. Change this if
%needed for lateral dynamics!

%Vinf_s is squared already
Rbh = [cos(ainf) 0 -sin(ainf);0 1 0;sin(ainf) 0 cos(ainf)];

forces = Rbh*[-D; 0; -L]; %Only Longitudinal Dynamics
[FX, FY, FZ] = deal(forces(1), forces(2), forces(3));
moments = cross(Marm,[FX, FY, FZ]);
[MX, MY, MZ] = deal(moments(1), moments(2), moments(3));

== matlab function hydrofoil_sim_unified/Hydrofoil Craft/Hydrofoil Forces/Hydrofoil [A]/STRUT FP/lateralDamp ==
  data: h_sub input; strutK output; zs input; V input; p input; cs input; rho parameter
function strutK = strutrolldamp(h_sub, zs, V, p, cs, rho)

strutK = -0.5*rho*V*2*pi*p*cs*(zs.^3-(zs+0.1-h_sub).^3)*(1/3);

== matlab function hydrofoil_sim_unified/Hydrofoil Craft/Hydrofoil Forces/Hydrofoil [A]/CP and Submergence ==
  data: lx output; ly output; ac input; lz output; foil_arm input
function [lx,ly,lz] = CP_HSF(ac, foil_arm)
% This function will calculate the moment arm for the center of 
% pressure of a hydrofoil based on control deflection. 
% Used when the pivot point is different from the center of pressure, and
% set to the original foil CP defined in the params otherwise.



lx = foil_arm(1);
ly = foil_arm(2);
lz = foil_arm(3);

== matlab function hydrofoil_sim_unified/Hydrofoil Craft/Hydrofoil Forces/Hydrofoil [FS]/Force and Moment Calculation ==
  data: L input; D input; FX output; ainf input; FY output; FZ output; Marm input; MX output; MY output; MZ output
function [FX, FY, FZ, MX, MY, MZ] = HydrodynamicForces(L, D, ainf, Marm)


%%%%%%%%% ----------------- %%%%%%%%

% Vrel is :
% u+qz-ry  
% v+rx-pz
% w+py-qx

%Inflow velocity is this vector's magnitude, however, in 2D analysis,
%considering the y direction velocity will lead to issues. Change this if
%needed for lateral dynamics!

%Vinf_s is squared already
Rbh = [cos(ainf) 0 -sin(ainf);0 1 0;sin(ainf) 0 cos(ainf)];

forces = Rbh*[-D; 0; -L]; %Only Longitudinal Dynamics
[FX, FY, FZ] = deal(forces(1), forces(2), forces(3));
moments = cross(Marm,[FX, FY, FZ]);
[MX, MY, MZ] = deal(moments(1), moments(2), moments(3));

== matlab function hydrofoil_sim_unified/Hydrofoil Craft/Hydrofoil Forces/Hydrofoil [FS]/STRUT FP/lateralDamp ==
  data: h_sub input; strutK output; zs input; V input; p input; cs input; rho parameter
function strutK = strutrolldamp(h_sub, zs, V, p, cs, rho)

strutK = -0.5*rho*V*2*pi*p*cs*(zs.^3-(zs+0.1-h_sub).^3)*(1/3);

== matlab function hydrofoil_sim_unified/sense/sonar/sensor/get_hs ==
  data: positionCG input size=[3 1]; h_s output size=1; euler_angles input size=[3 1]; sonar_position input size=[3 1]; d_s output size=[3 1]
function [h_s, d_s] = raycast(positionCG, euler_angles, sonar_position)


d_s = zeros(3,1);
h_s = (-positionCG(3) + sonar_position(1).*sin(euler_angles(2)) - ...
sonar_position(2).*cos(euler_angles(2)).*sin(euler_angles(1)) - ...
sonar_position(3).*cos(euler_angles(2)).*cos(euler_angles(1)))./(cos(euler_angles(2)).*cos(euler_angles(1)));

d_s(1) = sonar_position(1); 
d_s(2) = sonar_position(2); 
d_s(3) = h_s-sonar_position(3);

== matlab function hydrofoil_sim_unified/sense/sonar/getCGheight ==
  data: h_s input; height_measured output; DCM input; sonar_position input; height_filtered output size=[1]; bA parameter; bB parameter; bC parameter; bD parameter
function [height_measured, height_filtered]  = analyze_sonar(h_s, DCM, sonar_position, bA,bB, bC, bD)

% Persistent variables

persistent last_update_time fstate

NEDvector = DCM*[sonar_position(1); sonar_position(2); h_s+sonar_position(3)];
height_measured = -NEDvector(3); % flip sign

if isempty(last_update_time)
    last_update_time = -inf;

    fstate = (eye(size(bA))-bA)\(bB*height_measured);
end
fstate = bA*fstate+bB*height_measured;

height_filtered = bC*fstate+bD*height_measured;

== matlab function hydrofoil_sim_unified/sense/kalman_fusion ==
  data: sonarH input; Vgps input; z output size=[1]; u output size=[1]; accXZ input; w output size=[1]; angles input; deltat parameter
function [z,u,w] = state_estimate(sonarH, Vgps, accXZ, angles, deltat) 

%% implement z, u, w kalman estimator %%

%% Initialization
persistent P;
persistent xhat;
persistent yprev;

if isempty(P)
    xhat = [-0.3; 7; 0]; % initial guess
    P = diag([0.1,0.1,0.1]); 
end
if isempty(yprev)
    yprev = [0;0];
end



%% system model %%
dt = deltat;

theta = angles(2);

ymeas = [sonarH;Vgps];

A = [1, -dt * theta, dt; 0, 1, 0; 0, 0, 1];
B = [0 0; dt 0; 0 dt]; 
%% system model set %%

%Q =  diag([0.5*dt^2*(0.0132^2) dt*(0.0132^2) dt*(0.0132^2)]);
varu = (1.316*1e-2)^2;
varw = (1.316*1e-2)^2;
Q = 2*dt^2.*[varu*theta^2+varw, -varu*theta, varw;
            -varu*theta, varu, 0;
            varw, 0, varw];

R =  diag([0.03^2 0.05^2]);

u_in = accXZ; %[\dot{u};\dot{v}] acceleration as input

%% KF PREDICT %%
% this runs at 1/dt Hz 
[xhat, P] = kf_predict(xhat, P, u_in, Q);

%% KF UPDATE %%

% this only runs whenever new data comes
% sonar
if ymeas(1)~=yprev(1)
    H = [1 0 0];
    Rs = R(1,1);
    [xhat, P] = kf_update(ymeas(1), xhat, P, H, Rs);
    yprev(1) = ymeas(1);
end

% gps
if ymeas(2)~=yprev(2)
    H = [0 1 theta];
    Rs = R(2,2);
    [xhat, P] = kf_update(ymeas(2), xhat, P, H, Rs);
    yprev(2) = ymeas(2);
end

function [x_pred,P_pred] = kf_predict(x_in, P_in, u_input, Q)

    x_pred = A * x_in + B * u_input;
    P_pred = A * P_in * A' + Q;

end

function [x_up, P_up] = kf_update(y_meas, x_pred, P_pred, H, R)

    residual = y_meas-H*x_pred;
    K = P_pred*H'/(H*P_pred*H'+R);

    x_up = x_pred+K*residual;

    P_up = (eye(size(P_pred)) - K*H)*P_pred*(eye(size(P_pred))-K*H)'+K*R*K';

end

z = xhat(1);
u = xhat(2);
w = xhat(3);

end

== matlab function hydrofoil_sim_unified/Controller [Variant]/MPC-IP/Reference Previewer/MATLAB Function ==
  settings: updateMethod=DISCRETE  sampleTime=ts
  data: data parameter; seq output; steps parameter; t input; first output; next_t output
function [seq,first,next_t] = fcn(data,steps,t)
%#codegen
[seq,first,next_t] = mpcblock_preview('ref',data,steps,t);

== matlab function hydrofoil_sim_unified/Controller [Variant]/LPV-MPC-IDP/Reference Previewer/MATLAB Function ==
  settings: updateMethod=DISCRETE  sampleTime=ts
  data: data parameter; seq output; steps parameter; t input; first output; next_t output
function [seq,first,next_t] = fcn(data,steps,t)
%#codegen
[seq,first,next_t] = mpcblock_preview('ref',data,steps,t);

== matlab function hydrofoil_sim_unified/Controller [Variant]/LQI/Discrete LQRi no S//AW ==
  settings: updateMethod=DISCRETE
  data: reference input; states input; control_input output; u_trim input; Klqid parameter; Ka parameter; act_lims parameter
function control_input  = LQRi_discrete(reference, states,  u_trim, Klqid, Ka, act_lims)

% LQRi with internal sample-and-hold behavior
% Inputs:
%   u_ref   - feedforward/reference input
%   z_ref   - reference for tracking
%   y       - measured outputs (vector)
%   t       - current simulation time

% Parameters
T_s = 0.1;  % controller sample time

% Persistent variables
persistent xI_z xI_phi xI_theta
persistent last_update_time u_hold u_c

if isempty(last_update_time)
    xI_z = 0; xI_phi = 0; xI_theta = 0;
    last_update_time = -inf;
    u_c = zeros(3,1);
    u_hold = zeros(3,1);
end


states = states-reference;
% --- Tracking Errors ---
e_z = states(1);
e_phi = states(2);    
e_theta = states(3);  

% --- Integrate Error ---
xI_z = xI_z + T_s * e_z;
xI_phi = xI_phi + T_s * e_phi;
xI_theta = xI_theta + T_s * e_theta;

% --- Control Law ---
x_aug = [states; xI_z; xI_phi; xI_theta];

% Define gain K externally or inline
K = Klqid;  


% Compute control
u_c = u_trim - K * x_aug;


u_hold = u_c;



% --- Output ZOH value ---
control_input = u_hold;

== matlab function hydrofoil_sim_unified/Controller [Variant]/LQI-S/Discrete LQRi no AW ==
  settings: updateMethod=DISCRETE
  data: reference input; states input; control_input output; u_trim input; Klqid parameter; Ka parameter; act_lims parameter
function control_input  = LQRi_discrete(reference, states,  u_trim, Klqid, Ka, act_lims)

% LQRi with internal sample-and-hold behavior
% Inputs:
%   u_ref   - feedforward/reference input
%   z_ref   - reference for tracking
%   y       - measured outputs (vector)
%   t       - current simulation time

% Parameters
T_s = 0.1;  % controller sample time

% Persistent variables
persistent xI_z xI_phi xI_theta
persistent last_update_time u_hold u_c

if isempty(last_update_time)
    xI_z = 0; xI_phi = 0; xI_theta = 0;
    last_update_time = -inf;
    u_c = zeros(3,1);
    u_hold = zeros(3,1);
end


states = states-reference;
% --- Tracking Errors ---
e_z = states(1);
e_phi = states(2);    
e_theta = states(3);  

% --- Integrate Error ---
xI_z = xI_z + T_s * e_z ;
xI_phi = xI_phi + T_s * e_phi ;
xI_theta = xI_theta + T_s * e_theta ;

% --- Control Law ---
x_aug = [states; xI_z; xI_phi; xI_theta];

% Define gain K externally or inline
K = Klqid;  


% Compute control
u_c = u_trim - K * x_aug;

% this alone is saturation
u_hold = min(max(u_c, act_lims(:,1)), act_lims(:,2)); 



% --- Output ZOH value ---
control_input = u_hold;

== matlab function hydrofoil_sim_unified/Hydrofoil Craft/Hydrofoil Forces/Hydrofoil [A]/Foil Theory/AdditionalDrag/Additional Drag ==
  data: cdind input; dinc output; span input; hsub input; t input; c input; cdw output; cdint output; usted parameter
function [dinc, cdw, cdint]   = addedDrag(cdind, span, hsub, t, c, usted)

%V = 7m/s not very correct in general 
hsub = abs(hsub);
dinc = (2-(33*(hsub/span)^(3/2))/(33*(hsub/span)^(3/2)+1))*cdind;
frh = usted/sqrt(9.81*hsub);
cdw = 1/(2*frh^2)*(c/hsub)*exp(-2/frh^2);
cdint = 0.75*(t/c)-0.0003*(t/c)^(-2);

== matlab function hydrofoil_sim_unified/Controller [Variant]/LPV-MPC-IP/Reference Previewer/MATLAB Function ==
  settings: updateMethod=DISCRETE  sampleTime=ts
  data: data parameter; seq output; steps parameter; t input; first output; next_t output
function [seq,first,next_t] = fcn(data,steps,t)
%#codegen
[seq,first,next_t] = mpcblock_preview('ref',data,steps,t);
